simulink model "power_SVC"  (Simulink 6.0)
settings: Solver=ode23tb  StartTime=0.0  StopTime=1  MaxStep=1/60  RelTol=1e-4
undefined symbols (not defined in the file or in its folder): find_system, j
libraries: powerlib x10, powerlib_extras x2, simulink_extras x1
settings Model: Creator=by2815  LastModifiedBy=batserve  ExtModeAutoUpdateStatusClock=off
settings DataIOCC: SaveOutput=off  SaveTime=off  SignalLoggingName=sigsOut
settings DebuggingCC: CheckExecutionContextPreStartOutputMsg=on  CheckExecutionContextRuntimeOutputMsg=on  SolverPrmCheckMsg=none
settings HardwareCC: TargetUnknown=on

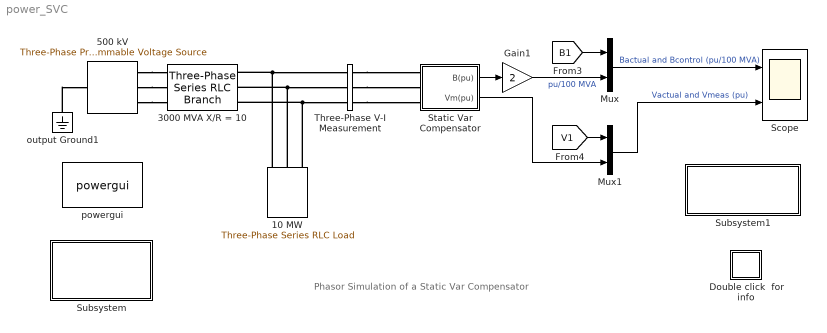
== system power_SVC ==
  note: Phasor Simulation of a Static Var Compensator
  10 MW : powerlib/Elements/Three-Phase Series RLC Load  Orientation=down  PhysicalDomain=powersysdomain  SubClassName=unknown  LeftPortType=p1  RightPortType=p1  LConnTagsString=A|B|C  Configuration=Y (grounded)  NominalVoltage=500e3  NominalFrequency=60  ActivePower=10e6  InductivePower=0  CapacitivePower=0  Measurements=None
  3000 MVA X/R = 10 : powerlib/Elements/Three-Phase Series RLC Branch  PhysicalDomain=powersysdomain  SubClassName=unknown  LeftPortType=p1  RightPortType=p1  LConnTagsString=A|B|C  RConnTagsString=A|B|C  Resistance=500e3^2/3000e6/10  Inductance=500e3^2/3000e6/(2*pi*60)  Capacitance=inf  Measurements=None
  500 kV : powerlib/Electrical Sources/Three-Phase Programmable Voltage Source  PositiveSequence="[500e3  0 60]"  VariationEntity=Amplitude  VariationType=Table of time-amplitude pairs  VariationStep=0.5  VariationRate=10  VariationMagnitude=0.25  VariationFrequency=0.05  VariationTiming=[0 20]  VariationPhaseA=off  Amplitudes="[ 1  0.97  1.03  1]"  TimeValues="[ 0  0.1 0.4  0.7]"  HarmonicGeneration=off  HarmonicA=[3 0.2 -25 0]  HarmonicB=[2 0.15 35 2]  Timing="[0.05  3]"
  Double click  for info : Subsystem
      mask Display: disp('?')
  Gain1 : Gain  Gain=2  SaturateOnIntegerOverflow=on
  Mux : Mux  Inputs=2
  Mux1 : Mux  Inputs=2
  Scope : Scope  NumInputPorts=2
      settings: TimeRange=1  YMin=-1~0.96  YMax=1~1.08
  Static Var Compensator : Subsystem  AncestorBlock=powerlib/Phasor Elements/Static Var Compensator  LoadFcn=find_system(gcs,'FollowLinks', 'on', 'LookUnderMasks', 'all');  mask(Static Var Compensator (Phasor Type)){mode=Voltage regulation, Vnom=500e3, Qnom=[200e6  -100e6], Pbase=200e6, Vref=1.0, Xs=0.03, Kp_Ki=[0  300], Bref=0.5, Tm=8e-3, Td=4e-3}
      mask prompts: mode "Mode of operation"; Vnom "Nominal voltage (Vrms Ph-Ph):"; Qnom "Reactive power limits [Qc(var>0)  Ql(var<0)]:"; Pbase "Three-phase base power Pbase (VA):"; Vref "Reference voltage Vref  (pu):"; Xs "Droop Xs (pu/Pbase):"; Kp_Ki "Voltage regulator [Kp(puB/puV)  Ki(puB/puV/s)]:"; Bref "Bref  for var control mode (pu/Pbase):"; Tm "Time constant of voltage measurement system Tm (s):"; Td "Average time delay due to thyristor valves firing Td (s):"
      mask help:
      | This block implements a  phasor model of a three-phase, three-wire Static Var Compensator (SVC).
      |
      | The B output signal (SVC susceptance in pu/Pbase)  is the output of the voltage regulator or the reference susceptance Bref in var control mode.
      | The Vm output is the measured positive-sequence voltage (pu).
      mask init:
      | Qc_nom=Qnom(1);
      | Ql_nom=Qnom(2);
      | Bmax=Qc_nom/Pbase;
      | Bmin=Ql_nom/Pbase;
      | Vbase=Vnom/sqrt(3)*sqrt(2);
      | Ibase=Pbase/Vnom/sqrt(3)*sqrt(2);
      | Kp=Kp_Ki(1);
      | Ki=Kp_Ki(2);;
      settings: CloseFcn=%3phaseVImeasurement
      mask Help: web(psbhelp)
      mask StyleString: popup(Voltage regulation|Var control (Fixed susceptance Bref)),edit,edit,edit,edit,edit,edit,edit,edit,edit
      mask CallbackString: powericon('psbcallbacks',gcb,'SVCblock');|||||||||
  Subsystem : Subsystem
      mask Display: disp('Signal Processing')
  Subsystem1 : Subsystem
      settings: OpenFcn=|
      | open('power_SVC.fig')
      | if exist('I1_imag') & exist('V1')
      |   hold on
      |    plot(-I1_imag,V1)
      | end
      mask Display: disp('Double click\nto plot\nV-I characteristic')
  Three-Phase V-I Measurement : powerlib/Measurements/Three-Phase V-I Measurement  VoltageMeasurement=phase-to-ground  SetLabelV=on  LabelV=Vabc  Vpu=on  Vbase=500e3  CurrentMeasurement=yes  SetLabelI=on  LabelI=Iabc  Ipu=on  Pbase=100e6  OutputType=Complex  PhasorSimulation=on  PSBequivalent=0
  output Ground1 : powerlib/Elements/Ground  Orientation=down  PhysicalDomain=powersysdomain  SubClassName=unknown  LeftPortType=p1  RightPortType=p1  LConnTagsString=a
  powergui : powerlib/powergui  Priority=2  Frange=[0:2:500]  Ylog=off  Xlog=on  save=off  variable=ZData  ZoomFFT=on  StartTime=0.0  cycles=1  DisplayStyle=1  fundamental=60  FreqAxis=off  MaxFrequency=1000  frequencyindice=1  frequencyindicesteady=1  RmsSteady=1  display=off  Ts=0  methode=on  frequency=60  echomessages=on
  wires:
  Mux/1 -> Scope/1  "Bactual and Bcontrol (pu/100 MVA)"
  Static Var Compensator/1(B(pu)) -> Gain1/1
  [B1] -> Mux/1
  Mux1/1 -> Scope/2  "Vactual and Vmeas (pu)"
  Static Var Compensator/2(Vm(pu)) -> Mux1/2
  [V1] -> Mux1/1
  Gain1/1 -> Mux/2  "pu/100 MVA"
  connections:
  output Ground1/LConn1 -- 500 kV/LConn1
  10 MW/LConn1 -- 3000 MVA X/R = 10/RConn1 -- Three-Phase V-I Measurement/LConn1
  10 MW/LConn2 -- 3000 MVA X/R = 10/RConn2 -- Three-Phase V-I Measurement/LConn2
  Three-Phase V-I Measurement/RConn1 -- Static Var Compensator/LConn1
  Three-Phase V-I Measurement/RConn2 -- Static Var Compensator/LConn2
  Three-Phase V-I Measurement/RConn3 -- Static Var Compensator/LConn3
  10 MW/LConn3 -- 3000 MVA X/R = 10/RConn3 -- Three-Phase V-I Measurement/LConn3
  500 kV/RConn1 -- 3000 MVA X/R = 10/LConn1
  500 kV/RConn2 -- 3000 MVA X/R = 10/LConn2
  500 kV/RConn3 -- 3000 MVA X/R = 10/LConn3

== system power_SVC/Double click  for info ==
  note: Demonstration
  note: 1. Dynamic response of the SVC
  note: The Three-Phase Programmable Voltage Source is used to vary the system voltage and observe the SVC performance. Initially the source is generating nominal voltage.
      | Then, voltage is successively decreased (0.97 pu at t = 0.1 s), increased (1.03 pu at t = 0.4 s)  and finally returned to nominal voltage (1 pu at t = 0.7 s).
      |
      | Start the simulation and observe  the SVC dynamic response to voltage steps on the Scope.
      | Trace 1 shows the actual  positive-sequence susceptance B1  and control signal output B of the voltage regulator.
      | Trace 2 shows the actual system positive-sequence voltage V1 and output Vm of the SVC measurement system.
      |
      | The SVC response speed depends on the voltage regulator integral gain Ki (Proportional gain Kp is set to zero), system strength (reactance Xn) and droop (reactance Xs).
      | If the voltage measurement time constant Tm and average time delay Td due to valve firing are neglected, the system can be approximated by a first order system
      | having a  closed loop time constant :
      |
      |     Tc= 1/(Ki*(Xn+Xs))
      |
      | With given system parameters (Ki = 300; Xn = 0.0667 pu/200 MVA; Xs = 0.03 pu/200 MVA), Tc = 0.0345 s. If you increase the regulator gain or decrease the system strength,
      | Tm and Td will non longer be negligible and you will observe an oscillatory response and eventually unstability.
  note: G. Sybille (Hydro-Quebec)
  note: A static var compensator (SVC) is used to regulate voltage on a 500 kV, 3000 MVA sytem. When system voltage is low the SVC generates reactive power
      | (SVC capacitive). When system voltage is high it absorbs reactive power (SVC inductive). The SVC is rated +200 Mvar capacitive and 100 Mvar inductive.
      | The Static Var Compensator block is a a phasor model  representing SVC static and dynamic characteristic at the system fundamental frequency.
      |
      | Open the SVC block menu and look at  its parameters. The SVC is set in voltage regulation mode with a reference voltage Vref=1.0 pu.
      | The voltage droop is 0.03 pu/ 200MVA, so that the voltage varies from 0.97 pu to 1.015 pu when the SVC current goes from fully capacitive to fully inductive.
      | Double click now on the blue block to display  the SVC V-I characteristic.
      |
      | The actual SVC positive-sequence voltage (V1) and susceptance  (B1) are measured inside the 'Signal Processing' subsystem, using the complex voltages Vabc
      | and complex currents Iabc returned by the Three-Phase V-I Measurement block.
  note: Circuit Description
  note: This demonstration illustrates steady-state and dynamic performance of the static var compensator (SVC) phasor model
  note: 2. Measurement of steady-state V-I characteristic
  note: In order to measure the SVC steady-state V-I characteristic,  you will now program a slow variation of the source voltage.
      | Open the Programmable Voltage Source menu and change the "Type of Variation" parameter to "Modulation". The modulation parameters are set to apply
      | a sinusoidal variation of the positive-sequence voltage between 0.75 and 1.25 pu in 20 seconds.
      | In the Simulation->Simulation Parameters menu change the stop time to 20 s and restart  simulation. When simulation is completed, double click the blue block.
      | The theoretical V-I characteristic is displayed (in red) together with the measured characteristic (in blue).

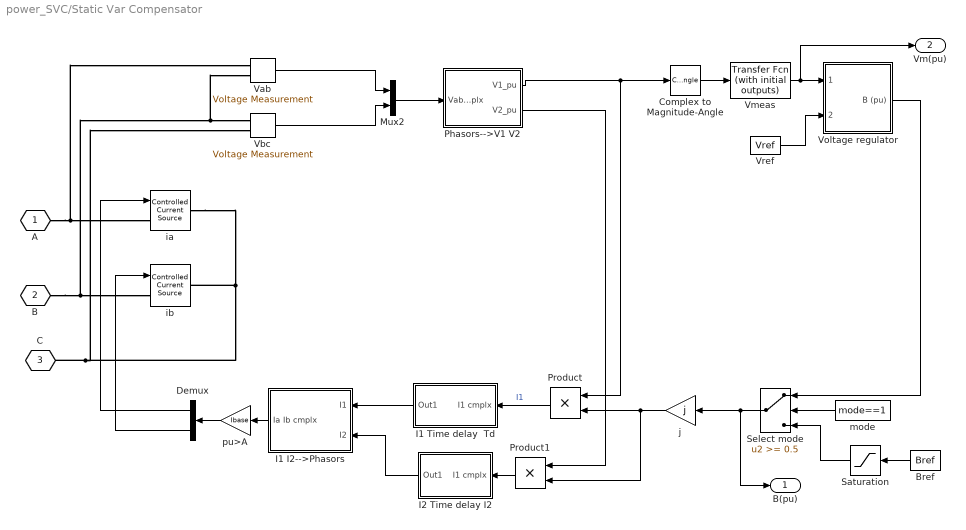
== system power_SVC/Static Var Compensator ==
  Bref : Constant  Orientation=left  Value=Bref
  Complex to Magnitude-Angle : ComplexToMagnitudeAngle  Output=Magnitude
  Demux : Demux  Orientation=left  Outputs=2
  I1 I2-->Phasors : Subsystem  Orientation=left
  I1 Time delay  Td : Subsystem  Orientation=left
  I2 Time delay I2 : Subsystem  Orientation=left
  Mux2 : Mux  Inputs=2
  Phasors-->V1 V2 : Subsystem
  Product : Product  Orientation=left  SaturateOnIntegerOverflow=on  InputSameDT=on
  Product1 : Product  Orientation=left  SaturateOnIntegerOverflow=on  InputSameDT=on
  Saturation : Saturate  Orientation=left  UpperLimit=Bmax  LowerLimit=Bmin
  Select mode : Switch  Orientation=left  Threshold=0.5  InputSameDT=on
  Vab : powerlib/Measurements/Voltage Measurement  PhasorSimulation=on  OutputType=Complex  PSBequivalent=0
  Vbc : powerlib/Measurements/Voltage Measurement  PhasorSimulation=on  OutputType=Complex  PSBequivalent=0
  Vmeas : simulink_extras/Additional Linear/Transfer Fcn (with initial outputs)  N=[1]  D="[Tm  1]"  Y0=Vref  U0=Vref
  Voltage regulator : Subsystem
  Vref : Constant  Value=Vref
  ia : powerlib/Electrical Sources/Controlled Current Source  Description=source block  Initialize=off  Amplitude=0  Phase=0  Frequency=0  Measurements=None
  ib : powerlib/Electrical Sources/Controlled Current Source  Description=source block  Initialize=off  Amplitude=0  Phase=0  Frequency=0  Measurements=None
  j : Gain  Orientation=left  Gain=j  SaturateOnIntegerOverflow=on
  mode : Constant  Orientation=left  Value=mode==1
  pu>A : Gain  Orientation=left  Gain=Ibase  SaturateOnIntegerOverflow=on
  A : PMIOPort  Port=1  Side=Left
  B : PMIOPort  Port=2  Side=Left
  C : PMIOPort  Port=3  Side=Left
  B(pu) : Outport
  Vm(pu) : Outport  Port=2
  wires:
  Product1/1 -> I2 Time delay I2/1(I1 cmplx)
  Phasors-->V1 V2/2(V2_pu) -> Product1/1
  j/1 -> Product1/2, Product/2
  Product/1 -> I1 Time delay  Td/1(I1 cmplx)  "I1"
  pu>A/1 -> Demux/1
  I1 Time delay  Td/1(Out1) -> I1 I2-->Phasors/1(I1)
  Vbc/1 -> Mux2/2
  Vab/1 -> Mux2/1
  Complex to Magnitude-Angle/1 -> Vmeas/1
  I2 Time delay I2/1(Out1) -> I1 I2-->Phasors/2(I2)
  I1 I2-->Phasors/1(Ia Ib cmplx) -> pu>A/1
  Vmeas/1 -> Vm(pu)/1, Voltage regulator/1(V1meas (pu))
  Vref/1 -> Voltage regulator/2(Vref (pu))
  Phasors-->V1 V2/1(V1_pu) -> Product/1, Complex to Magnitude-Angle/1
  Mux2/1 -> Phasors-->V1 V2/1(Vab Vbc cmplx)
  Select mode/1 -> j/1, B(pu)/1
  Bref/1 -> Saturation/1
  Voltage regulator/1(B (pu)) -> Select mode/1
  mode/1 -> Select mode/2
  Demux/1 -> ia/1
  Demux/2 -> ib/1
  Saturation/1 -> Select mode/3
  connections:
  A/RConn1 -- ia/LConn1 -- Vab/LConn1
  B/RConn1 -- ib/LConn1 -- Vbc/LConn1 -- Vab/LConn2
  ia/RConn1 -- ib/RConn1 -- C/RConn1 -- Vbc/LConn2

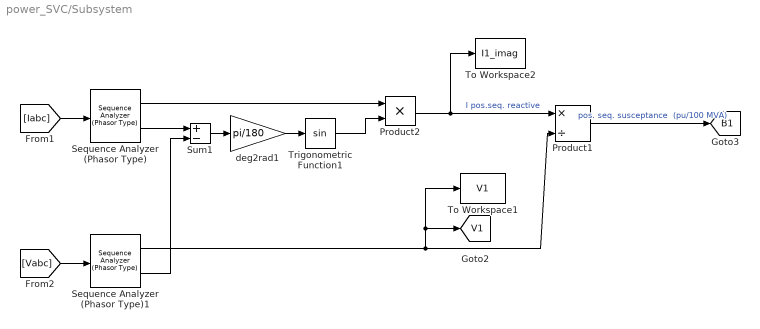
== system power_SVC/Subsystem ==
  Product1 : Product  Inputs=*/  SaturateOnIntegerOverflow=on
  Product2 : Product  Inputs=**  SaturateOnIntegerOverflow=on
  Sequence Analyzer (Phasor Type) : powerlib_extras/Phasor Library/Sequence Analyzer (Phasor Type)  seq=Positive
  Sequence Analyzer (Phasor Type)1 : powerlib_extras/Phasor Library/Sequence Analyzer (Phasor Type)  seq=Positive
  Sum1 : Sum  Inputs=+-  SaturateOnIntegerOverflow=on
  To Workspace1 : ToWorkspace  VariableName=V1  SampleTime=-1  SaveFormat=Array
  To Workspace2 : ToWorkspace  VariableName=I1_imag  SampleTime=-1  SaveFormat=Array
  Trigonometric Function1 : Trigonometry
  deg2rad1 : Gain  Gain=pi/180  SaturateOnIntegerOverflow=on
  tag scope: B1=global, V1=global
  wires:
  Sequence Analyzer (Phasor Type)1/1 -> Product1/2, To Workspace1/1, [V1]
  Product1/1 -> [B1]  "pos. seq. susceptance  (pu/100 MVA)"
  [Iabc] -> Sequence Analyzer (Phasor Type)/1
  [Vabc] -> Sequence Analyzer (Phasor Type)1/1
  Sum1/1 -> deg2rad1/1
  deg2rad1/1 -> Trigonometric Function1/1
  Sequence Analyzer (Phasor Type)1/2 -> Sum1/2
  Sequence Analyzer (Phasor Type)/2 -> Sum1/1
  Sequence Analyzer (Phasor Type)/1 -> Product2/1
  Trigonometric Function1/1 -> Product2/2
  Product2/1 -> Product1/1, To Workspace2/1  "I pos.seq. reactive"

== system power_SVC/Subsystem1 ==

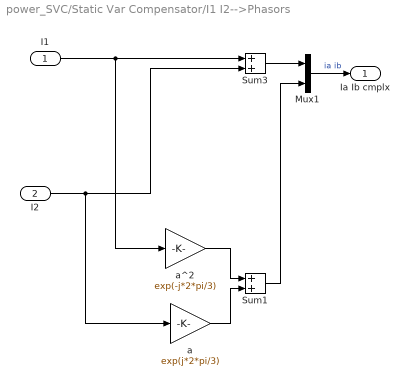
== system power_SVC/Static Var Compensator/I1 I2-->Phasors ==
  I1 : Inport  Port=1  LatchInput=off
  I2 : Inport  Port=2  LatchInput=off
  Mux1 : Mux  Inputs=2
  Sum1 : Sum  SaturateOnIntegerOverflow=on  InputSameDT=on
  Sum3 : Sum  SaturateOnIntegerOverflow=on  InputSameDT=on
  a : Gain  Gain=exp(j*2*pi/3)  SaturateOnIntegerOverflow=on
  a^2 : Gain  Gain=exp(-j*2*pi/3)  SaturateOnIntegerOverflow=on
  Ia Ib cmplx : Outport
  wires:
  I1/1 -> a^2/1, Sum3/1
  I2/1 -> a/1, Sum3/2
  a^2/1 -> Sum1/1
  a/1 -> Sum1/2
  Sum3/1 -> Mux1/1
  Sum1/1 -> Mux1/2
  Mux1/1 -> Ia Ib cmplx/1  "ia ib"

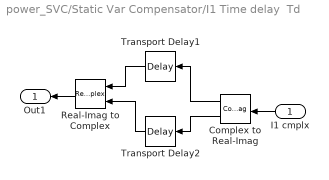
== system power_SVC/Static Var Compensator/I1 Time delay  Td ==
  I1 cmplx : Inport  Orientation=left  Port=1  LatchInput=off
  Complex to Real-Imag : ComplexToRealImag  Orientation=left
  Real-Imag to Complex : RealImagToComplex  Orientation=left
  Transport Delay1 : TransportDelay  Orientation=left  DelayTime=Td
  Transport Delay2 : TransportDelay  Orientation=left  DelayTime=Td
  Out1 : Outport  Orientation=left
  wires:
  Transport Delay2/1 -> Real-Imag to Complex/2
  Transport Delay1/1 -> Real-Imag to Complex/1
  Complex to Real-Imag/2 -> Transport Delay2/1
  Complex to Real-Imag/1 -> Transport Delay1/1
  Real-Imag to Complex/1 -> Out1/1
  I1 cmplx/1 -> Complex to Real-Imag/1

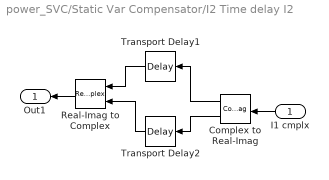
== system power_SVC/Static Var Compensator/I2 Time delay I2 ==
  I1 cmplx : Inport  Orientation=left  Port=1  LatchInput=off
  Complex to Real-Imag : ComplexToRealImag  Orientation=left
  Real-Imag to Complex : RealImagToComplex  Orientation=left
  Transport Delay1 : TransportDelay  Orientation=left  DelayTime=Td
  Transport Delay2 : TransportDelay  Orientation=left  DelayTime=Td
  Out1 : Outport  Orientation=left
  wires:
  I1 cmplx/1 -> Complex to Real-Imag/1
  Real-Imag to Complex/1 -> Out1/1
  Complex to Real-Imag/1 -> Transport Delay1/1
  Complex to Real-Imag/2 -> Transport Delay2/1
  Transport Delay1/1 -> Real-Imag to Complex/1
  Transport Delay2/1 -> Real-Imag to Complex/2

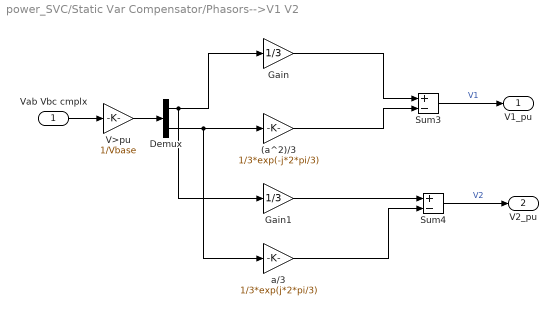
== system power_SVC/Static Var Compensator/Phasors-->V1 V2 ==
  Vab Vbc cmplx : Inport  Port=1  LatchInput=off
  (a^2)/3 : Gain  Gain=1/3*exp(-j*2*pi/3)  SaturateOnIntegerOverflow=on
  Demux : Demux  Outputs=2
  Gain : Gain  Gain=1/3  SaturateOnIntegerOverflow=on
  Gain1 : Gain  Gain=1/3  SaturateOnIntegerOverflow=on
  Sum3 : Sum  Inputs=+-  SaturateOnIntegerOverflow=on  InputSameDT=on
  Sum4 : Sum  Inputs=+-  SaturateOnIntegerOverflow=on  InputSameDT=on
  V>pu : Gain  Gain=1/Vbase  SaturateOnIntegerOverflow=on
  a/3 : Gain  Gain=1/3*exp(j*2*pi/3)  SaturateOnIntegerOverflow=on
  V1_pu : Outport
  V2_pu : Outport  Port=2
  wires:
  V>pu/1 -> Demux/1
  Sum3/1 -> V1_pu/1  "V1"
  Demux/1 -> Gain1/1, Gain/1
  a/3/1 -> Sum4/2
  Gain1/1 -> Sum4/1
  Vab Vbc cmplx/1 -> V>pu/1
  Gain/1 -> Sum3/1
  Demux/2 -> a/3/1, (a^2)/3/1
  (a^2)/3/1 -> Sum3/2
  Sum4/1 -> V2_pu/1  "V2"

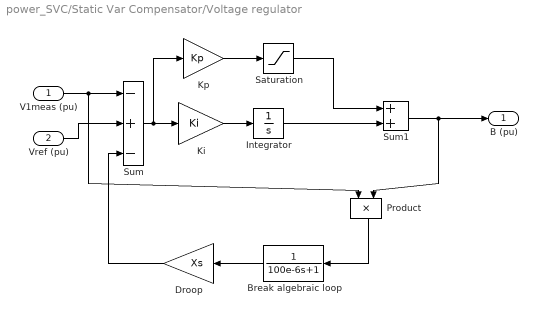
== system power_SVC/Static Var Compensator/Voltage regulator ==
  V1meas (pu) : Inport  Port=1  LatchInput=off
  Vref (pu) : Inport  Port=2  LatchInput=off
  Break algebraic loop : TransferFcn  Orientation=left  Denominator=[100e-6 1]
  Droop : Gain  Orientation=left  Gain=Xs  SaturateOnIntegerOverflow=on
  Integrator : Integrator  LimitOutput=on  UpperSaturationLimit=Bmax  LowerSaturationLimit=Bmin
  Ki : Gain  Gain=Ki  SaturateOnIntegerOverflow=on
  Kp : Gain  Gain=Kp  SaturateOnIntegerOverflow=on
  Product : Product  Orientation=down  SaturateOnIntegerOverflow=on  InputSameDT=on
  Saturation : Saturate  UpperLimit=Bmax  LowerLimit=Bmin
  Sum : Sum  Inputs=-+-  SaturateOnIntegerOverflow=on  InputSameDT=on
  Sum1 : Sum  SaturateOnIntegerOverflow=on
  B (pu) : Outport  InitialOutput=0
  wires:
  Break algebraic loop/1 -> Droop/1
  Droop/1 -> Sum/3
  V1meas (pu)/1 -> Product/1, Sum/1
  Ki/1 -> Integrator/1
  Vref (pu)/1 -> Sum/2
  Sum/1 -> Ki/1, Kp/1
  Product/1 -> Break algebraic loop/1
  Kp/1 -> Saturation/1
  Integrator/1 -> Sum1/2
  Saturation/1 -> Sum1/1
  Sum1/1 -> B (pu)/1, Product/2
